simulink model "SMC_sim_CSEI"  (R2022a)
settings: Solver=ode4  StartTime=0.0  StopTime=T_final  FixedStep=Ts  RelTol=1e-3
values from neighbouring files (symbols this model uses):
  BL = [20 10 10]    [ASMC_ESO_sim_CSEI_Scripts.m]    (also in ASMC_FTESO_sim_CSEI_Scripts.m; SMC_ESO_sim_CSEI_Scripts.m; SMC_sim_CSEI_Scripts.m)
  Control_allocation = 1    [ASMC_ESO_sim_CSEI_Scripts.m]    (also in ASMC_FTESO_sim_CSEI_Scripts.m; SMC_ESO_sim_CSEI_Scripts.m; SMC_sim_CSEI_Scripts.m)
  current = [0;0]    [ASMC_ESO_sim_CSEI_Scripts.m]    (also in ASMC_FTESO_sim_CSEI_Scripts.m; Berthing_Control_PID_CSEI_Scripts.m; Position_Control_PID_CSEI_Scripts.m; Position_Control_PID_CSEI_Scripts_released.m)
  K_SMC = [20 20 50]    [ASMC_ESO_sim_CSEI_Scripts.m]    (also in ASMC_FTESO_sim_CSEI_Scripts.m; SMC_ESO_sim_CSEI_Scripts.m; SMC_sim_CSEI_Scripts.m)
  lamda = [5.0 5.0 10]    [ASMC_ESO_sim_CSEI_Scripts.m]    (also in ASMC_FTESO_sim_CSEI_Scripts.m; SMC_ESO_sim_CSEI_Scripts.m; SMC_sim_CSEI_Scripts.m)
  option = 0    [ASMC_ESO_sim_CSEI_Scripts.m]    (also in ASMC_FTESO_sim_CSEI_Scripts.m; SMC_ESO_sim_CSEI_Scripts.m = 1; SMC_sim_CSEI_Scripts.m = 1)
  psi_ref = 40    [ASMC_ESO_sim_CSEI_Scripts.m]    (also in ASMC_FTESO_sim_CSEI_Scripts.m; SMC_ESO_sim_CSEI_Scripts.m; SMC_sim_CSEI_Scripts.m)
  tau_max = 20*[3; 3; 3]    [ASMC_ESO_sim_CSEI_Scripts.m]    (also in ASMC_FTESO_sim_CSEI_Scripts.m; SMC_ESO_sim_CSEI_Scripts.m; SMC_sim_CSEI_Scripts.m)
  u0 = [0 1.52021873594 0.0130499995288]    [trimout.mat]
  v_max = 10    [ASMC_ESO_sim_CSEI_Scripts.m]    (also in ASMC_FTESO_sim_CSEI_Scripts.m; Position_Control_PID_CSEI_Scripts.m = 2; Position_Control_PID_CSEI_Scripts_released.m = 2; SMC_ESO_sim_CSEI_Scripts.m)
  w_d = 0.5    [ASMC_ESO_sim_CSEI_Scripts.m]    (also in ASMC_FTESO_sim_CSEI_Scripts.m; SMC_ESO_sim_CSEI_Scripts.m; SMC_sim_CSEI_Scripts.m)
  x0 = zeros(6,1)    [Berthing_Control_PID_CSEI_Scripts.m]    (also in Position_Control_PID_CSEI_Scripts.m; Position_Control_PID_CSEI_Scripts_released.m; Waypoint_Control_PID_CSEI_Scripts.m; Waypoint_Control_PID_CSEI_Scripts_LLA.m)
  x_ref = 7    [ASMC_ESO_sim_CSEI_Scripts.m]    (also in ASMC_FTESO_sim_CSEI_Scripts.m; SMC_ESO_sim_CSEI_Scripts.m; SMC_sim_CSEI_Scripts.m)
  y_ref = 7    [ASMC_ESO_sim_CSEI_Scripts.m]    (also in ASMC_FTESO_sim_CSEI_Scripts.m; SMC_ESO_sim_CSEI_Scripts.m; SMC_sim_CSEI_Scripts.m)
  zeta_d = 1    [ASMC_ESO_sim_CSEI_Scripts.m]    (also in ASMC_FTESO_sim_CSEI_Scripts.m; SMC_ESO_sim_CSEI_Scripts.m; SMC_sim_CSEI_Scripts.m)
libraries: simulink_extras x3
settings Model: Creator=ADMIN  LastModifiedBy=ADMIN

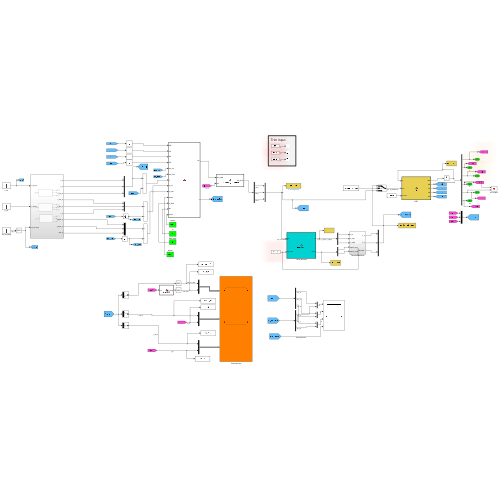
[thumbnail: Simulink's stored preview of the top-level diagram]
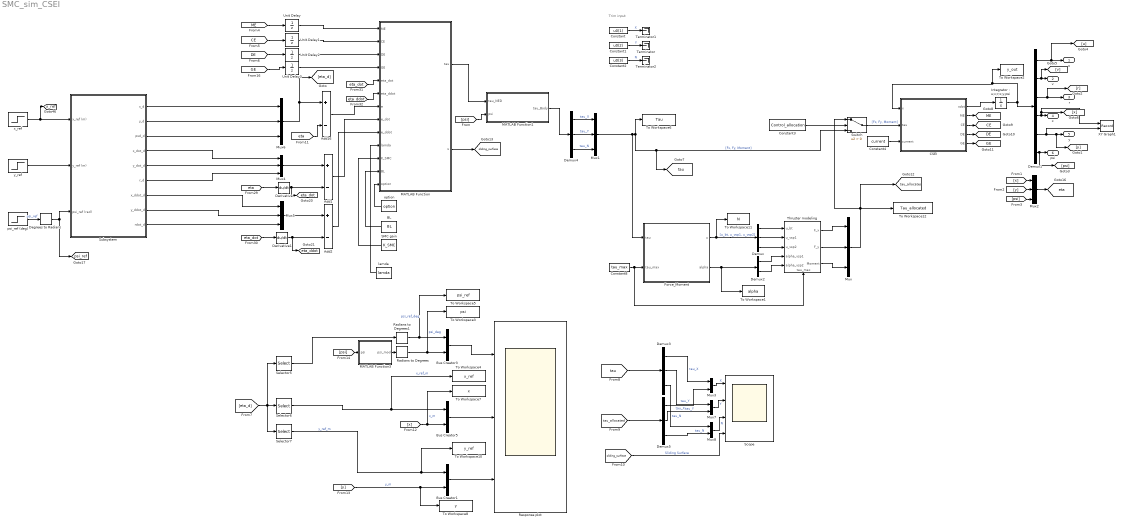
== system SMC_sim_CSEI ==
  note: Trim input
  Add1 : Sum  Inputs=+-
  Add16 : Sum  Inputs=+-
  Add2 : Sum  Inputs=+-
  BL : Constant  Value=BL
  Bus Creator1 : BusCreator  Inputs=2
  Bus Creator3 : BusCreator  Inputs=2
  Bus Creator5 : BusCreator  Inputs=2
  CSEI : MATLAB Function  TreatAsAtomicUnit=on
  Constant : Constant  Value=u0(1)
  Constant1 : Constant  Value=u0(2)
  Constant2 : Constant  Value=u0(3)
  Constant3 : Constant  Value=Control_allocation
  Constant4 : Constant  Value=current
  Constant8 : Constant  Value=tau_max
  Degrees to Radians : simulink_extras/Transformations/Degrees to Radians
  Demux{,3..5} (4 alike) : Demux  Outputs=3
  Demux1 : Demux  Outputs=6
  Demux2 : Demux  Outputs=2
  Derivative : Derivative
  Derivative1 : Derivative
  Force_Moment : MATLAB Function  TreatAsAtomicUnit=on
  "Integrator : u;v;r;x;y;psi" : Integrator  InitialCondition=x0
  MATLAB Function : MATLAB Function  TreatAsAtomicUnit=on
  MATLAB Function1 : MATLAB Function  TreatAsAtomicUnit=on
  MATLAB Function3 : MATLAB Function  TreatAsAtomicUnit=on
  Mux{,1..2,4..6} (6 alike) : Mux  Inputs=3
  Mux3 : Mux  Inputs=2
  Mux7 : Mux  Inputs=2
  Mux8 : Mux  Inputs=2
  Radians to Degrees : simulink_extras/Transformations/Radians to Degrees
  Radians to Degrees1 : simulink_extras/Transformations/Radians to Degrees
  Response plot : Scope  NumInputPorts=3
  SMC gain : Constant  Value=K_SMC
  Scope : Scope  NumInputPorts=4
  Selector5 : Selector  InputPortWidth=3  IndexOptions=Index vector (dialog)  Indices=[3]  OutputSizes=1
  Selector6 : Selector  InputPortWidth=3  IndexOptions=Index vector (dialog)  Indices=[1]  OutputSizes=1
  Selector7 : Selector  InputPortWidth=3  IndexOptions=Index vector (dialog)  Indices=[2]  OutputSizes=1
  Subsystem : Subsystem
  Switch : Switch  Criteria=u2 > Threshold  SaturateOnIntegerOverflow=off  InputSameDT=off
  Terminator : Terminator
  Terminator1 : Terminator
  Terminator2 : Terminator
  Thruster modeling : Subsystem
      settings: PortSchema="{\"entries\":[{\"content\":{\"sides\":[{\"content\":{\"connectorIds\":[\"In1\",\"In2\",\"In3\",\"In4\",\"In5\"]},\"type\":\"ConnectorPlacement.EquallySpacedRectSide\",\"uuid\":\"a9c62c9e-2a2a-45d5-affb-b7e02571c4f5\"},{\"content\":{\"connectorIds\":[\"Out1\",\"Out2\",\"Out3\"],\"side\":\"RIGHT\"},\"type\":\"ConnectorPlacement.EquallySpacedRectSide\",\"uuid\":\"bfdff314-1a15-4488-bfde-1b5f82948245\"},{\"content\":{\"connectorIds\":[],\"side\":\"TOP\"},\"type\":\"ConnectorPlacement.EquallySpacedRectSide\",\"uuid\":\"bddef62a-91eb-4612-9a88-29ec8ace0b5e\"},{\"content\":{\"connectorIds\":[\"In6\"],\"side\":\"BOTTOM\"},\"type\":\"ConnectorPlacement.EquallySpacedRectSide\",\"uuid\":\"97d017d6-0e26-4257-956b-3bb507a639f3\"}]},\"type\":\"ConnectorPlacement.EquallySpacedConnector\",\"uuid\":\"a9966a75-95cf-4066-83e4-2624c4c1c778\"}],\"packageUris\":[\"http://schema.mathworks.com/mf0/Connector/R2020b\"],\"version\":\"1.0\"}"
  To Workspace1 : ToWorkspace  VariableName=alpha  SampleTime=-1
  To Workspace10 : ToWorkspace  VariableName=y_ref  SampleTime=-1
  To Workspace11 : ToWorkspace  VariableName=N  SampleTime=-1
  To Workspace12 : ToWorkspace  VariableName=Tau_allocated  SampleTime=-1
  To Workspace2 : ToWorkspace  VariableName=y_out  SampleTime=-1
  To Workspace3 : ToWorkspace  VariableName=psi  SampleTime=-1
      settings: Save2DSignal=2-D array (concatenate along first dimension)
  To Workspace4 : ToWorkspace  VariableName=x_ref  SampleTime=-1
  To Workspace5 : ToWorkspace  VariableName=psi_ref  SampleTime=-1
  To Workspace6 : ToWorkspace  VariableName=Tau  SampleTime=-1
  To Workspace7 : ToWorkspace  VariableName=x  SampleTime=-1
      settings: Save2DSignal=2-D array (concatenate along first dimension)
  To Workspace8 : ToWorkspace  VariableName=y  SampleTime=-1
  Unit Delay{,1..3} (4 alike) : UnitDelay  SampleTime=-1  HasFrameUpgradeWarning=on
  XY Graph1 : Record  FileSettingsInternal="{\"entries\":[{\"content\":{\"excelSettings\":{\"content\":{},\"type\":\"Streamout.ExcelSettings\"}},\"type\":\"Streamout.FileSettingStorage\",\"uuid\":\"f2668684-e551-420c-8344-7084dbd290d9\"}],\"packageUris\":[\"http://schema.mathworks.com/mf0/streamout_blocks/R2020a\"],\"version\":\"1.0\"}"  Layout=[1 1]  SignalsInternal="{\"entries\":[{\"content\":{\"signals\":[{\"content\":{\"blockPath\":[\"SMC_sim_CSEI/XY Graph1\"],\"channel\":[],\"dimensions\":[1],\"domain\":\"SMC_sim_CSEI/XY Graph1\",\"lineColor\":\"#a2142f\",\"plots\":[],\"port\":1,\"sid\":[\"\"],\"signalID\":5899,\"signalName\":\"Demux1:4\"},\"type\":\"RecordBlkView.Signal\",\"uuid\":\"32d1aa87-d3de-4197-8e3b-0b7511eb53a1\"},{\"content\":{\"blockPath\":[\"SMC_sim_CSEI/XY Graph1\"],\"channel\":[],\"dimensions\":[1],\"domain\":\"SMC_sim_CSEI/XY Graph1\",\"lineColor\":\"#139fff\",\"plots\":[],\"port\":2,\"sid\":[\"\"],\"signalID\":5903,\"signalName\":\"Demux1:5\"},\"type\":\"RecordBlkView.Signal\",\"uuid\":\"b039884d-20c5-413c-b660-524e60067f55\"}]},\"type\":\"RecordBlkView.InputSignals\",\"uuid\":\"fa957d13-001a-4b01-b8f6-a09f36e62a29\"}],\"packageUris\":[\"http://schema.mathworks.com/mf0/streamout_blocks/R2020a\"],\"version\":\"1.0\"}"  VisualizationBindings="{\"xyplotplugin\":{\"info\":[{\"series\":[],\"subplotID\":1}]}}"  CompatibilityTag=XY
  lamda : Constant  Value=lamda
  option : Constant  Value=option
  psi_ref (deg) : Step  Time=10  After=psi_ref  SampleTime=0
  x_ref : Step  Time=5  After=x_ref  SampleTime=0
  y_ref : Step  Time=5  After=y_ref  SampleTime=0
  u : Outport  VectorParamsAs1DForOutWhenUnconnected=off
  v : Outport  Port=2  VectorParamsAs1DForOutWhenUnconnected=off
  r : Outport  Port=3  VectorParamsAs1DForOutWhenUnconnected=off
  x : Outport  Port=4  VectorParamsAs1DForOutWhenUnconnected=off
  y : Outport  Port=5  VectorParamsAs1DForOutWhenUnconnected=off
  psi : Outport  Port=6  VectorParamsAs1DForOutWhenUnconnected=off
  tag scope: CE=global, DE=global, GE=global, ME=global, eta=global, eta_ddot=global, eta_dot=global, psi_ref=global, sliding_surface=global, tau=global, tau_allocated=global, x_ref=global
  wires:
  Demux1/2 -> [v], v/1
  Demux1/4 -> [x], XY Graph1/1, x/1
  Demux1/3 -> [r], r/1
  CSEI/1(xdot) -> "Integrator : u;v;r;x;y;psi"/1
  Demux1/6 -> [psi], psi/1
  Demux1/1 -> [u], u/1
  Demux1/5 -> XY Graph1/2, [y], y/1
  Mux1/1 -> Force_Moment/1(tau), [tau], Switch/3, To Workspace6/1  "[Fx, Fy, Moment]"
  Force_Moment/1(u) -> Demux/1, To Workspace11/1  "[u_bt, u_vsp1, u_vsp2]"
  Constant3/1 -> Switch/2
  Constant1/1 -> Terminator/1  "Y"
  Constant/1 -> Terminator1/1  "X"
  Constant2/1 -> Terminator2/1  "N"
  Constant4/1 -> CSEI/3(current)
  Demux/1 -> Thruster modeling/1(u_bt)
  Demux/2 -> Thruster modeling/2(u_vsp1)
  Demux/3 -> Thruster modeling/3("u_vsp2 ")
  Force_Moment/2(alpha) -> To Workspace1/1, Demux2/1
  Demux2/1 -> Thruster modeling/4(alpha_vsp1)
  Demux2/2 -> Thruster modeling/5(alpha_vsp2)
  Thruster modeling/1(F_x) -> Mux/1
  Thruster modeling/2(F_y) -> Mux/2
  Thruster modeling/3("Moment ") -> Mux/3
  Mux/1 -> [tau_allocated], To Workspace12/1, Switch/1
  Constant8/1 -> Thruster modeling/6(tau_max), Force_Moment/2(tau_max)
  CSEI/2(ME) -> [ME]
  CSEI/3(CE) -> [CE]
  CSEI/4(DE) -> [DE]
  MATLAB Function/1(tau) -> MATLAB Function1/1(tau_NED)
  [GE] -> Unit Delay3/1
  Add16/1 -> MATLAB Function/7(e)
  [psi] -> MATLAB Function1/2(psi)
  Add2/1 -> MATLAB Function/9(e_ddot)
  Derivative1/1 -> [eta_ddot], Add2/2
  [eta_ddot] -> MATLAB Function/6(eta_ddot)
  SMC gain/1 -> MATLAB Function/11(K_SMC)
  x_ref/1 -> [x_ref], Subsystem/1(x_ref (m))
  Derivative/1 -> [eta_dot], Add1/2
  [DE] -> Unit Delay2/1
  [eta_dot] -> MATLAB Function/5(eta_dot)
  [eta] -> Derivative/1
  Subsystem/2(y_d) -> Mux6/2
  Subsystem/1(x_d) -> Mux6/1
  Mux4/1 -> Add1/1
  [CE] -> Unit Delay1/1
  [ME] -> Unit Delay/1
  Subsystem/4(x_dot_d) -> Mux4/1
  Subsystem/5(y_dot_d) -> Mux4/2
  y_ref/1 -> Subsystem/2(y_ref (m))
  lamda/1 -> MATLAB Function/10(lamda)
  Subsystem/8(y_ddot_d) -> Mux5/2
  Degrees to Radians/1 -> Subsystem/3(psi_ref (rad)), [psi_ref]
  Add1/1 -> MATLAB Function/8(e_dot)
  Subsystem/7(x_ddot_d) -> Mux5/1
  Subsystem/9(rdot_d) -> Mux5/3
  [eta_dot] -> Derivative1/1
  psi_ref (deg)/1 -> Degrees to Radians/1  "psi_ref"
  Subsystem/6(r_d) -> Mux4/3
  Subsystem/3(psd_d) -> Mux6/3
  Mux6/1 -> [eta_d], Add16/1
  [eta] -> Add16/2
  Mux5/1 -> Add2/1
  BL/1 -> MATLAB Function/12(BL)
  Demux4/1 -> Mux1/1  "tau_X"
  Demux4/2 -> Mux1/2  "tau_Y"
  Demux4/3 -> Mux1/3  "tau_N"
  CSEI/5(GE) -> [GE]
  [x] -> Mux2/1
  [y] -> Mux2/2
  [psi] -> Mux2/3
  Mux2/1 -> [eta]
  [x] -> Bus Creator5/2, To Workspace7/1  "x_m"
  Bus Creator1/1 -> Response plot/3
  Bus Creator3/1 -> Response plot/1
  [psi] -> MATLAB Function3/1(psi)
  [y] -> To Workspace8/1, Bus Creator1/2  "y_m"
  MATLAB Function3/1(psi_mod) -> Radians to Degrees/1
  Radians to Degrees1/1 -> To Workspace5/1, Bus Creator3/1  "psi_ref_deg"
  Selector5/1 -> Radians to Degrees1/1
  Radians to Degrees/1 -> Bus Creator3/2, To Workspace3/1  "psi_deg"
  Selector7/1 -> To Workspace10/1, Bus Creator1/1  "y_ref_m"
  [eta_d] -> Selector5/1, Selector6/1, Selector7/1
  Bus Creator5/1 -> Response plot/2
  Selector6/1 -> To Workspace4/1, Bus Creator5/1  "x_ref_m"
  "Integrator : u;v;r;x;y;psi"/1 -> Demux1/1, CSEI/1(x), To Workspace2/1
  MATLAB Function1/1(tau_Body) -> Demux4/1
  Switch/1 -> CSEI/2(tau)  "[Fx, Fy, Moment]"
  [tau] -> Demux3/1
  [tau_allocated] -> Demux5/1
  Mux3/1 -> Scope/1  "X"
  Mux8/1 -> Scope/3  "N"
  Demux3/1 -> Mux3/1  "tau_X"
  Demux3/2 -> Mux7/1  "tau_Y"
  Demux3/3 -> Mux8/1  "tau_N"
  Demux5/1 -> Mux3/2  "tau_X"
  Demux5/2 -> Mux7/2  "tau_Y"
  Demux5/3 -> Mux8/2  "tau_N"
  Mux7/1 -> Scope/2  "Y"
  option/1 -> MATLAB Function/13(option)
  MATLAB Function/2(s) -> [sliding_surface]
  [sliding_surface] -> Scope/4  "Sliding Surface"
  Unit Delay/1 -> MATLAB Function/1(ME)
  Unit Delay1/1 -> MATLAB Function/2(CE)
  Unit Delay2/1 -> MATLAB Function/3(DE)
  Unit Delay3/1 -> MATLAB Function/4(GE)

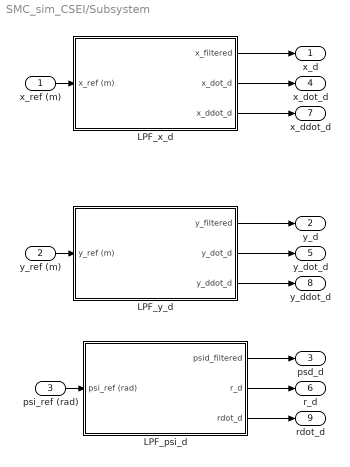
== system SMC_sim_CSEI/Subsystem ==
  x_ref (m) : Inport
  y_ref (m) : Inport  Port=2
  psi_ref (rad) : Inport  Port=3
  LPF_psi_d : Subsystem
  LPF_x_d : Subsystem
  LPF_y_d : Subsystem
  x_d : Outport
  y_d : Outport  Port=2
  psd_d : Outport  Port=3
  x_dot_d : Outport  Port=4
  y_dot_d : Outport  Port=5
  r_d : Outport  Port=6
  x_ddot_d : Outport  Port=7
  y_ddot_d : Outport  Port=8
  rdot_d : Outport  Port=9
  wires:
  LPF_x_d/3(x_ddot_d) -> x_ddot_d/1
  LPF_x_d/2(x_dot_d) -> x_dot_d/1
  LPF_y_d/1(y_filtered) -> y_d/1
  x_ref (m)/1 -> LPF_x_d/1(x_ref (m))
  psi_ref (rad)/1 -> LPF_psi_d/1(psi_ref (rad))
  LPF_y_d/2(y_dot_d) -> y_dot_d/1
  LPF_x_d/1(x_filtered) -> x_d/1
  LPF_psi_d/2(r_d) -> r_d/1
  y_ref (m)/1 -> LPF_y_d/1(y_ref (m))
  LPF_psi_d/1(psid_filtered) -> psd_d/1
  LPF_psi_d/3(rdot_d) -> rdot_d/1
  LPF_y_d/3(y_ddot_d) -> y_ddot_d/1

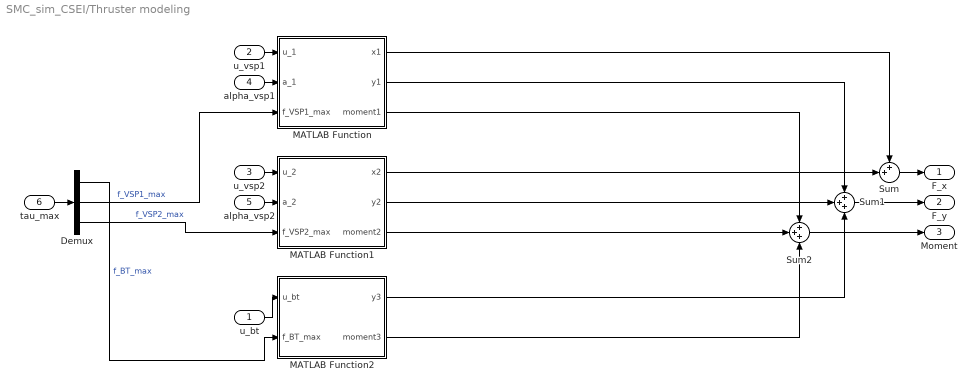
== system SMC_sim_CSEI/Thruster modeling ==
  u_bt : Inport
  u_vsp1 : Inport  Port=2
  "u_vsp2 " : Inport  Port=3
  alpha_vsp1 : Inport  Port=4
  alpha_vsp2 : Inport  Port=5
  tau_max : Inport  Port=6
  Demux : Demux  Outputs=3
  MATLAB Function : MATLAB Function  TreatAsAtomicUnit=on
  MATLAB Function1 : MATLAB Function  TreatAsAtomicUnit=on
  MATLAB Function2 : MATLAB Function  TreatAsAtomicUnit=on
  Sum : Sum  Inputs=++|
  Sum1 : Sum  Inputs=+++
  Sum2 : Sum  Inputs=+++
  F_x : Outport
  F_y : Outport  Port=2
  "Moment " : Outport  Port=3
  wires:
  u_bt/1 -> MATLAB Function2/1(u_bt)
  alpha_vsp2/1 -> MATLAB Function1/2(a_2)
  u_vsp1/1 -> MATLAB Function/1(u_1)
  "u_vsp2 "/1 -> MATLAB Function1/1(u_2)
  MATLAB Function1/1(x2) -> Sum/2
  Sum/1 -> F_x/1
  Sum1/1 -> F_y/1
  MATLAB Function1/2(y2) -> Sum1/2
  MATLAB Function2/1(y3) -> Sum1/3
  Sum2/1 -> "Moment "/1
  MATLAB Function2/2(moment3) -> Sum2/3
  MATLAB Function1/3(moment2) -> Sum2/2
  MATLAB Function/3(moment1) -> Sum2/1
  MATLAB Function/1(x1) -> Sum/1
  MATLAB Function/2(y1) -> Sum1/1
  tau_max/1 -> Demux/1
  Demux/1 -> MATLAB Function2/2(f_BT_max)  "f_BT_max"
  alpha_vsp1/1 -> MATLAB Function/2(a_1)
  Demux/2 -> MATLAB Function/3(f_VSP1_max)  "f_VSP1_max"
  Demux/3 -> MATLAB Function1/3(f_VSP2_max)  "f_VSP2_max"

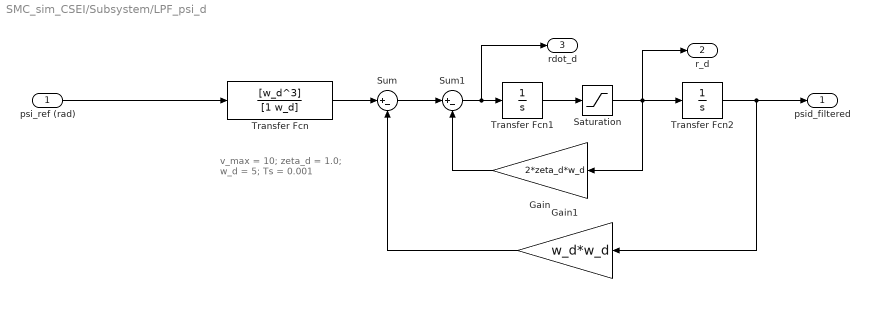
== system SMC_sim_CSEI/Subsystem/LPF_psi_d ==
  note: v_max = 10;
      | zeta_d = 1.0;
      | w_d = 5;
      | Ts = 0.001
  psi_ref (rad) : Inport
  Gain : Gain  Gain=2*zeta_d*w_d
  Gain1 : Gain  Gain=w_d*w_d
  Saturation : Saturate  UpperLimit=v_max  LowerLimit=-v_max  LinearizeAsGain=off
  Sum : Sum  Inputs=|+-
  Sum1 : Sum  Inputs=|+-
  Transfer Fcn : TransferFcn  Numerator=[w_d^3]  Denominator=[1 w_d]
  Transfer Fcn1 : TransferFcn  Denominator=[1 0]
  Transfer Fcn2 : TransferFcn  Denominator=[1 0]
  psid_filtered : Outport
  r_d : Outport  Port=2
  rdot_d : Outport  Port=3
  wires:
  Transfer Fcn/1 -> Sum/1
  Transfer Fcn1/1 -> Saturation/1
  Sum1/1 -> rdot_d/1, Transfer Fcn1/1
  Saturation/1 -> r_d/1, Gain/1, Transfer Fcn2/1
  Gain1/1 -> Sum/2
  Sum/1 -> Sum1/1
  Transfer Fcn2/1 -> psid_filtered/1, Gain1/1
  Gain/1 -> Sum1/2
  psi_ref (rad)/1 -> Transfer Fcn/1

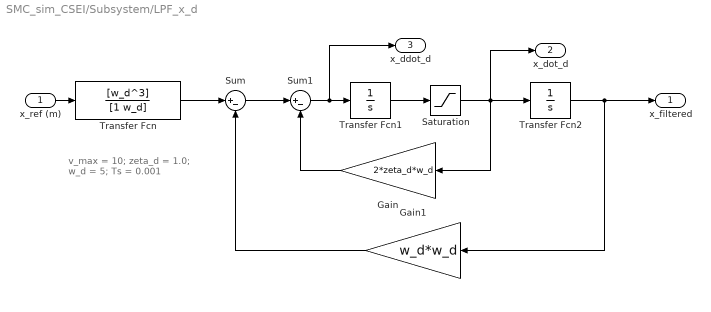
== system SMC_sim_CSEI/Subsystem/LPF_x_d ==
  note: v_max = 10;
      | zeta_d = 1.0;
      | w_d = 5;
      | Ts = 0.001
  x_ref (m) : Inport
  Gain : Gain  Gain=2*zeta_d*w_d
  Gain1 : Gain  Gain=w_d*w_d
  Saturation : Saturate  UpperLimit=v_max  LowerLimit=-v_max  LinearizeAsGain=off
  Sum : Sum  Inputs=|+-
  Sum1 : Sum  Inputs=|+-
  Transfer Fcn : TransferFcn  Numerator=[w_d^3]  Denominator=[1 w_d]
  Transfer Fcn1 : TransferFcn  Denominator=[1 0]
  Transfer Fcn2 : TransferFcn  Denominator=[1 0]
  x_filtered : Outport
  x_dot_d : Outport  Port=2
  x_ddot_d : Outport  Port=3
  wires:
  Transfer Fcn/1 -> Sum/1
  Transfer Fcn1/1 -> Saturation/1
  Sum1/1 -> x_ddot_d/1, Transfer Fcn1/1
  Saturation/1 -> x_dot_d/1, Gain/1, Transfer Fcn2/1
  Gain1/1 -> Sum/2
  Sum/1 -> Sum1/1
  Transfer Fcn2/1 -> x_filtered/1, Gain1/1
  Gain/1 -> Sum1/2
  x_ref (m)/1 -> Transfer Fcn/1

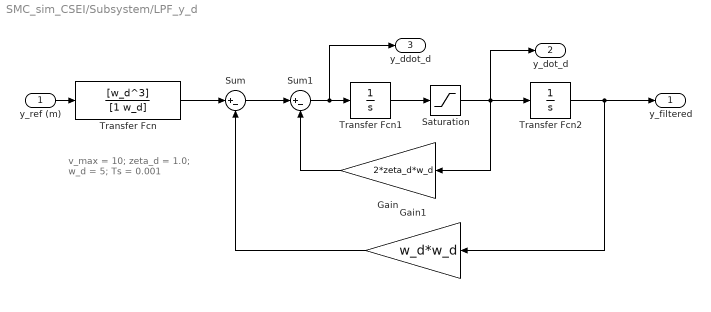
== system SMC_sim_CSEI/Subsystem/LPF_y_d ==
  note: v_max = 10;
      | zeta_d = 1.0;
      | w_d = 5;
      | Ts = 0.001
  y_ref (m) : Inport
  Gain : Gain  Gain=2*zeta_d*w_d
  Gain1 : Gain  Gain=w_d*w_d
  Saturation : Saturate  UpperLimit=v_max  LowerLimit=-v_max  LinearizeAsGain=off
  Sum : Sum  Inputs=|+-
  Sum1 : Sum  Inputs=|+-
  Transfer Fcn : TransferFcn  Numerator=[w_d^3]  Denominator=[1 w_d]
  Transfer Fcn1 : TransferFcn  Denominator=[1 0]
  Transfer Fcn2 : TransferFcn  Denominator=[1 0]
  y_filtered : Outport
  y_dot_d : Outport  Port=2
  y_ddot_d : Outport  Port=3
  wires:
  Transfer Fcn/1 -> Sum/1
  Transfer Fcn1/1 -> Saturation/1
  Sum1/1 -> y_ddot_d/1, Transfer Fcn1/1
  Saturation/1 -> y_dot_d/1, Gain/1, Transfer Fcn2/1
  Gain1/1 -> Sum/2
  Sum/1 -> Sum1/1
  Transfer Fcn2/1 -> y_filtered/1, Gain1/1
  Gain/1 -> Sum1/2
  y_ref (m)/1 -> Transfer Fcn/1

== matlab function SMC_sim_CSEI/Force_Moment ==
  data: tau input; u output; alpha output; tau_max input
function [u, alpha] = force2input(tau, tau_max)
    % Mapping of desired force (tau) to input to the actuators (u)
    % Input: 3DOF desired forces and moment in body-frame, tau = [X Y N]'
    % Output: input signals to the actuators, u = [u_BT u_VSP1 u_VSP2]';
    %         angles of the two VSPs, alpha = [alpha_VSP1 alpha_VSP2]';
    %         angular rates of the VSPs, omega = [omega_VSP1 omega_VSP2]'
    %
    % Author: Caroline Fleischer, Elias Gauslaa, Jakob Jensen
    % Date:   20.02.2020

%% Initializing values
    ly_VSP = 0.055;         % Moment arm along y for VSP
    lx_VSP = 0.4574;        % Moment arm along x for VSP
    lx_BT = 0.3875;         % Moment arm along x for BT
    
    % default
%     f_VSP1_max = 0.45;      % Max thrust VSP1 
%     f_VSP2_max = 0.45;      % Max thrust VSP2
%     f_BT_max = 0.3;         % Max thrust BT
%     
    % test
    f_VSP1_max = tau_max(2);      % Max thrust VSP1
    f_VSP2_max = tau_max(3);      % Max thrust VSP2
    f_BT_max = tau_max(1);         % Max thrust BT

%     omega_VSP1 = 0.199;     % Rotation speed for VSP1, LABORATORY ONLY
%     omega_VSP2 = 0.235;     % Rotation speed for VSP2, LABORATORY ONLY
    alpha = zeros(2,1);     % VSP angles
%     omega = zeros(2,1);     % VSP angular rates
    u = zeros(3,1);         % Input vector to the VSPs and BT

    B = [  1      0       1      0      0;
           0      1       0      1      1;
         ly_VSP -lx_VSP -ly_VSP -lx_VSP lx_BT]; % Configuration matrix
%% Thrust allocation
    B_dagger = pinv(B);                         % Calculating dagger

    %f_vps1,x f_vps1,y, 
    f_cmd = B_dagger*tau;                       % Forces and moment

    u_cmd = [norm(f_cmd(1:2))/f_VSP1_max;
             norm(f_cmd(3:4))/f_VSP2_max;
             f_cmd(5)/f_BT_max];                % Calculating input to each
                                                % thruster

    % Saturation: Limit input signal to VSPs to be within [0,1]
    if u_cmd(1) < 0
        u_cmd(1) = 0;
    elseif u_cmd(1) > 1
        u_cmd(1) = 1;
    else
        u_cmd(1) = u_cmd(1);
    end

    if u_cmd(2) < 0
        u_cmd(2) = 0;
    elseif u_cmd(2) > 1
        u_cmd(2) = 1;
    else
        u_cmd(2) = u_cmd(2);
    end

    % Saturation: Limit input signal to BT to be within [-1,1]
    if u_cmd(3) < -1
        u_cmd(3) = -1;
    elseif u_cmd(3) > 1
        u_cmd(3) = 1;
    else
        u_cmd(3) = u_cmd(3);
    end
    
    alpha(1) = atan2(f_cmd(2),f_cmd(1));         % Calculate angle of VSP1
    alpha(2) = atan2(f_cmd(4),f_cmd(3));         % Calculate angle of VSP2
    
%     omega(1) = omega_VSP1;                       % Output omega LAB ONLY
%     omega(2) = omega_VSP2;                       % Output omega LAB ONLY

    BT_gain = 1;                                 % Gain used in LAB

    u(1) = u_cmd(3)*BT_gain;                     % Output input to BT
    u(2) = u_cmd(1);                             % Output input to VSP1
    u(3) = u_cmd(2);                             % Output input to VSP2
    
end

== matlab function SMC_sim_CSEI/MATLAB Function ==
  data: ME input; tau output; CE input; DE input; GE input; eta_dot input; eta_ddot input; e input; e_dot input; e_ddot input; lamda input; K_SMC input; BL input; option input; s output
function [tau, s] = SMC(ME, CE, DE, GE, eta_dot, eta_ddot, e, e_dot, e_ddot, lamda, K_SMC, BL, option)


%  u:     surge velocity          (m/s)
%  v:     sway velocity           (m/s)
%  w:     heave velocity          (m/s)
%  p:     roll velocity           (rad/s)
%  q:     pitch velocity          (rad/s)
%  r:     yaw velocity            (rad/s)
%  x:     position in x direction (m)
%  y:     position in y direction (m)
%  z:     position in z direction (m)
%  phi:   roll angle              (rad)
%  theta: pitch angle             (rad)
%  psi:   yaw angle               (rad)


s = e_dot + lamda.*e;
s_dot = e_ddot + lamda.*e_dot;

tau_eq = ME*(eta_ddot+s_dot)+(CE+DE)*(eta_dot+s)+GE;

if option == 1
    tau_sw = K_SMC.*tanh(s./BL);

else
    tau_sw = K_SMC.*sign(s);
end


tau = tau_eq + tau_sw;

== matlab function SMC_sim_CSEI/MATLAB Function3 ==
  data: psi input; psi_mod output
function psi_mod = wrapToPi(psi)

psi_mod = mod(psi + pi, 2*pi) - pi;

== matlab function SMC_sim_CSEI/CSEI ==
  data: xdot output; x input; tau input; current input; ME output; CE output; DE output; GE output
function [xdot, ME, CE, DE, GE]  = CSEI(x, tau, current)
%% nu = [u, v, r], eta = [x, y, psi]
%  u:     surge velocity          (m/s)
%  v:     sway velocity           (m/s)
%  r:     yaw velocity            (rad/s)
%  x:     position in x direction (m)
%  y:     position in y direction (m)
%  psi:   yaw angle               (rad)

% This block calculates the change in position and heading given the
% current position and heading and velocities.


% State and current variables
nu = x(1:3); eta = x(4:6);
%% Initializing parameters
R = [cos(eta(3)) -sin(eta(3)) 0;
     sin(eta(3)) cos(eta(3)) 0;
     0 0 1];                        % Rotation matrix with heading
nu_c = R'*[current;0];              % Current velocity vector in body frame
nu_r = nu-nu_c;                     % Relative velocity
u   = nu_r(1);                      % Speed in x
v   = nu_r(2);                      % Speed in y
r   = nu_r(3);                      % Yaw rate

tau = [tau(1);tau(2);tau(3)];
%% MATRICES 
m    = 14.11;   I_z  =  1.7600;   x_g = 0.0375;

%% Added mass
X_ud  =     -2.0;											
					Y_vd =      -10.0;	N_vd =    -0.0;		
					Y_rd =      -0.0;	N_rd =    -1.0;	

%% Total mass matrix
m_11 = m-X_ud;
m_22 = m-Y_vd;
m_23 = m*x_g-Y_rd;
m_32 = m*x_g-N_vd;
m_33 = I_z-N_rd;

M    = [m_11 0    0
        0    m_22 m_23
        0    m_32 m_33];
	
%% Damping coefficients
% Comments at the end of the lines indicate the old values used.
X_u		= -0.6555;		X_v		= 0;
X_uu 	= 0.3545;		X_vv	= -2.443;
X_uuu 	= -3.787;		X_vvv	= 0;

						Y_v		= -1.33; 			Y_r		= -7.250; 
						Y_vv	= -2.776;			Y_rr	= -3.450; 
						Y_vvv	= -64.91;			Y_rrr	= 0;
						
						Y_rv	= -0.805;			Y_vr	= -0.845;

						N_v		= 0;				N_r		= -1.900;
						N_vv	= -0.2088;			N_rr	= -0.750;
						N_vvv	= 0;				N_rrr	= 0;
						
						N_rv	= 0.130;			N_vr	= 0.080;

%% Correolis matrix
c_13 = -(m-Y_vd)*v-(m*x_g-Y_rd)*r;
c_23 = (m-X_ud)*u;
C    = [0     0     c_13
        0     0     c_23
        -c_13 -c_23 0   ];

%% Assembly of the damping matrix
d_11 = -X_u - X_uu*u - X_uuu*u^2;
d_22 = -Y_v - Y_vv*v - Y_vvv*v^2 - Y_rv*abs(r);
d_33 = -N_r - N_rr*abs(r) - N_rrr*r^2 - N_vr*abs(v);

d_12 = -X_v - X_vv*v - X_vvv*v^2;
d_23 = -Y_r - Y_rr*abs(r) - Y_rrr*r^2 - Y_vr*abs(v);
d_32 = -N_v - N_vv*v - N_vvv*v^2 - N_rv*abs(r);

D    = [d_11 0 0
        0    d_22 d_23
        0    d_32 d_33];

%% Initializing
psi = eta(3);                       % Heading
R = [cos(psi) -sin(psi) 0
     sin(psi) cos(psi)  0
     0        0         1];         % Rotation matrix with heading
 
%% Calculating
eta_dot = R*(nu);
%% CALCULATION
nu_dot = M\(tau-(C+D)*nu_r);
tau_curr = (C+D)*nu_c;
xdot = [nu_dot;  % u, v, r
        eta_dot]; % x, y, psi

R_diff = [-sin(psi)*r -cos(psi)*r  0;
           cos(psi)*r  -sin(psi)*r  0;
           0         0         0];
inv_R = [ cos(psi), sin(psi), 0;
        -sin(psi), cos(psi), 0;
          0, 0, 1];                 
ME = R*M*inv_R;
CE = R*(C-M*inv_R*R_diff)*inv_R;
DE = R*D*inv_R;
GE = 0;
end

== matlab function SMC_sim_CSEI/MATLAB Function1 ==
  data: tau_NED input; tau_Body output; psi input
function tau_Body = Coordinate_Conversion(tau_NED, psi)

R = [cos(psi), -sin(psi), 0;
     sin(psi), cos(psi), 0;
      0, 0, 1];

tau_Body = inv(R)*tau_NED;

== matlab function SMC_sim_CSEI/Thruster modeling/MATLAB Function ==
  data: x1 output size=1; y1 output size=1; u_1 input size=1; a_1 input size=1; moment1 output size=1; f_VSP1_max input
function [x1,y1,moment1] = fcn(u_1, a_1, f_VSP1_max)
% This function takes in the input to VSP1 and calculates the resulting
% forces and moment.
    ly_VSP = 0.055;                         % Moment arm along y
    lx_VSP = 0.4574;                        % Moment arm along x
%     f_VSP1_max = 0.45;                      % Max thrust available
%     f_VSP1_max = 2.5;                      % Max thrust available

x1 = u_1*f_VSP1_max*cos(a_1);               % Resulting forces in x
y1 = u_1*f_VSP1_max*sin(a_1);               % Resulting forces in y
moment1 = x1*ly_VSP*(1) + y1*lx_VSP*(-1);   % Resulting moment

== matlab function SMC_sim_CSEI/Thruster modeling/MATLAB Function1 ==
  data: x2 output size=1; u_2 input size=1; y2 output size=1; a_2 input size=1; moment2 output size=1; f_VSP2_max input
function [x2,y2,moment2] = fcn(u_2,a_2, f_VSP2_max)
% This function takes in the input to VSP2 and calculates the resulting
% forces and moment.
    ly_VSP = 0.055;                         % Moment arm along y
    lx_VSP = 0.4574;                        % Moment arm along x
%     f_VSP2_max = 0.45;                      % Max thrust available
%     f_VSP2_max = 2.5;                      % Max thrust available

x2 = u_2*f_VSP2_max*cos(a_2);               % Resulting forces in x
y2 = u_2*f_VSP2_max*sin(a_2);               % Resulting forces in y
moment2 = x2*ly_VSP*(-1) + y2*lx_VSP*(-1);  % Resulting moment

== matlab function SMC_sim_CSEI/Thruster modeling/MATLAB Function2 ==
  data: u_bt input size=1; y3 output size=1; moment3 output size=1; f_BT_max input
function [y3,moment3] = fcn(u_bt, f_BT_max)
% This function takes in the input to the BT and calculates the resulting
% forces and moment.
    lx_BT = 0.3875;         % Moment arm along x
%     f_BT_max = 0.3;         % Max thrust available
%     f_BT_max = 2;         % Max thrust available
    
    y3 = u_bt*f_BT_max;     % Resulting force in y
    moment3 = y3*lx_BT;     % Resulting moment
